simulink model "FuzzyPIConScenario2"  (Simulink 9.3)
settings: Solver=VariableStepAuto  StartTime=0.0  StopTime=20.0  RelTol=1e-3
undefined symbols (not defined in the file or in its folder): sigbuilder_block
libraries: fuzblock x1
settings Model: LogicAnalyzerSignalOrdering=6826ba55-d383-4eb1-a829-21d225758932,556b48ee-a90b-40eb-b5dc-605fc91328ef,eba38db0-7cbc-4169-bdcd-0de638f60d3a  Creator=Kostas  LastModifiedBy=Kostas
settings DataIOCC: SaveFormat=Dataset  SignalLoggingSaveFormat=Dataset  ReturnWorkspaceOutputs=on
settings OptimizationCC: LifeSpan=auto
settings DebuggingCC: UnderspecifiedInitializationDetection=Simplified  MergeDetectMultiDrivingBlocksExec=error  FcnCallInpInsideContextMsg=error  SFUnexpectedBacktrackingDiag=error  SFNoUnconditionalDefaultTransitionDiag=error  SFExecutionAtInitializationDiag=warning  ArithmeticOperatorsInVariantConditions=error
settings HardwareCC: ProdBitPerPointer=64  ProdBitPerSizeT=64  ProdBitPerPtrDiffT=64  ProdLargestAtomicFloat=Float  ProdIntDivRoundTo=Zero  ProdEndianess=LittleEndian  ProdWordSize=64  ProdHWDeviceType=Intel->x86-64 (Windows64)
settings ModelReferenceCC: PropagateSignalLabelsOutOfModel=on
settings SFSimCC: SimUseLocalCustomCode=on
settings RTWCC: RTWUseLocalCustomCode=on
settings CodeAppCC: StateflowObjectComments=off
settings GRTTargetCC: TargetLangStandard=C99 (ISO)  CombineOutputUpdateFcns=on  GRTInterface=off
settings ConfigComp: CovMetricSettings=dwe  CovHtmlReporting=off  CovSaveCumulativeToWorkspaceVar=off  CovSaveSingleToWorkspaceVar=off  CovExternalEMLEnable=on

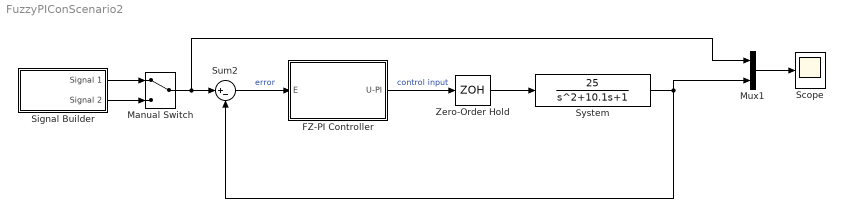
== system FuzzyPIConScenario2 ==
  FZ-PI Controller : Subsystem
  Manual Switch : ManualSwitch
  Mux1 : Mux  Inputs=2
  Scope : Scope
  Signal Builder : Subsystem  Tag=STV Subsys  LoadFcn=sigbuilder_block('load');  StartFcn=sigbuilder_block('start');  StopFcn=sigbuilder_block('stop');  ClipboardFcn=sigbuilder_block('clipboard');  mask(Sigbuilder block){tuvar=[0:10]}
      mask help: Simulink:masks:SigbuilderBlock_MD
      mask init:
      | if ~strcmp(get_param(bdroot(gcbh),'SimulationStatus'),'stopped') tuvar = sigbuilder_block('maskInit'); end
      settings: CopyFcn=sigbuilder_block('copy');  DeleteFcn=sigbuilder_block('delete');  ModelCloseFcn=sigbuilder_block('modelClose');  PreSaveFcn=sigbuilder_block('preSave');  PauseFcn=sigbuilder_block('pause');  ContinueFcn=sigbuilder_block('continue');  NameChangeFcn=sigbuilder_block('namechange');  OpenFcn=sigbuilder_block('open',[5.4 42.6 1141.2 444.6 ]);  CloseFcn=sigbuilder_block('close');
      mask Display: plot(0, 0, 100, 100,[2, 2, 32, 32, 2], [68, 8, 8, 68, 68],[32, 2], [38, 38], [32, 19, 2],[53, 60, 44], [32, 17, 17, 2],[16, 16, 31, 31]);txt = getActiveGroup(gcbh);text(2, 100, txt,'verticalAlignment', 'top');
  Sum2 : Sum  Inputs=|+-
  System : TransferFcn  Numerator=[25]  Denominator=[1 10.1 1]
  Zero-Order Hold : ZeroOrderHold  SampleTime=0.01
  wires:
  Zero-Order Hold/1 -> System/1
  FZ-PI Controller/1(U-PI) -> Zero-Order Hold/1  "control input"
  Sum2/1 -> FZ-PI Controller/1(E)  "error"
  System/1 -> Sum2/2, Mux1/2
  Mux1/1 -> Scope/1
  Manual Switch/1 -> Sum2/1, Mux1/1
  Signal Builder/2(Signal 2) -> Manual Switch/2
  Signal Builder/1(Signal 1) -> Manual Switch/1

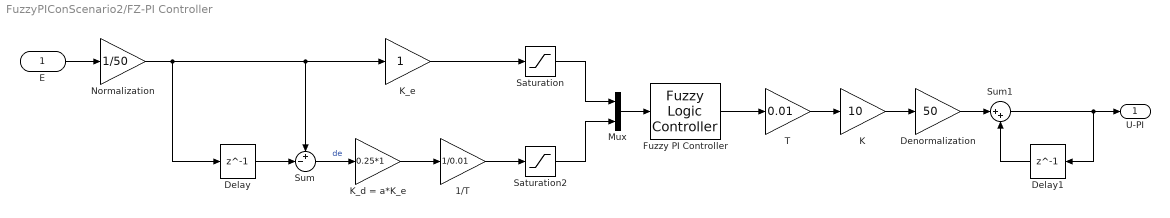
== system FuzzyPIConScenario2/FZ-PI Controller ==
  E : Inport
  1/T : Gain  Gain=1/0.01
  Delay : Delay  DelayLength=1  InitialCondition=0
  Delay1 : Delay  DelayLength=1  InitialCondition=0
  Denormalization : Gain  Gain=50
  Fuzzy PI Controller : fuzblock/Fuzzy Logic  Controller  FIS='fuzzyPIController.fis'  OutputSampleNumber=101  DataType=double  FuzzifiedInputs=off  RuleFiringStrengths=off  RuleOutputs=off  AggregatedOutputs=off  SimulateUsing=Interpreted execution  OutOfRangeInputValueMessage=warning  NoRuleFiredMessage=warning  EmptyOutputFuzzySetMessage=warning
  K : Gain  Gain=10
  K_d = a*K_e : Gain  Gain=0.25*1
  K_e : Gain
  Mux : Mux  Inputs=2
  Normalization : Gain  Gain=1/50
  Saturation : Saturate
  Saturation2 : Saturate
  Sum : Sum  Inputs=+-|
  Sum1 : Sum  Inputs=|++
  T : Gain  Gain=0.01
  U-PI : Outport
  wires:
  Saturation2/1 -> Mux/2
  Mux/1 -> Fuzzy PI Controller/1
  Saturation/1 -> Mux/1
  Sum1/1 -> Delay1/1, U-PI/1
  Delay1/1 -> Sum1/2
  K_d = a*K_e/1 -> 1/T/1
  Sum/1 -> K_d = a*K_e/1  "de"
  E/1 -> Normalization/1
  K_e/1 -> Saturation/1
  T/1 -> K/1
  Denormalization/1 -> Sum1/1
  Delay/1 -> Sum/2
  Fuzzy PI Controller/1 -> T/1
  1/T/1 -> Saturation2/1
  K/1 -> Denormalization/1
  Normalization/1 -> Delay/1, K_e/1, Sum/1

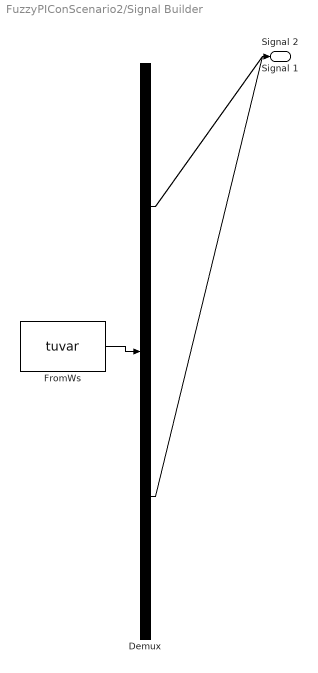
== system FuzzyPIConScenario2/Signal Builder ==
  Demux : Demux  Tag=STV Demux  Outputs=2
  FromWs : FromWorkspace  Tag=STV FromWs  VariableName=tuvar  SampleTime=0  SigBuilderData=DataTag0  VnvData=DataTag1
      SigBuilderData=|
      | common.afterFinalStr = 'Extrapolate'
      | common.sampleTime = 0
      | dataSet.timeRange = [0 20]
      | dataSet.name = 'Group 1'
      | sbobj.Groups.Name = 'Group 1'
      | sbobj.Groups.Signals(1).Name = 'Signal 1'
      | sbobj.Groups.Signals(1).XData = [0 5 5 10 10 20]
      | sbobj.Groups.Signals(1).YData = [50 50 20 20 40 40]
      | sbobj.Groups.Signals(2).Name = 'Signal 2'
      | sbobj.Groups.Signals(2).XData = [0 5 10 20]
      | sbobj.Groups.Signals(2).YData = [0 50 50 0]
      | sbobj.Groups.TimeRange = [0 20]
  Signal 1 : Outport  Tag=STV Outport
  Signal 2 : Outport  Tag=STV Outport  Port=2
  wires:
  FromWs/1 -> Demux/1
  Demux/1 -> Signal 1/1
  Demux/2 -> Signal 2/1
